simulink model "example_rotor_loop"  (R2016a)
settings: Solver=VariableStepAuto  StartTime=0.0  StopTime=20  RelTol=1e-3
libraries: simulink x2
settings Model: Creator=mgreiff  LastModifiedBy=mgreiff

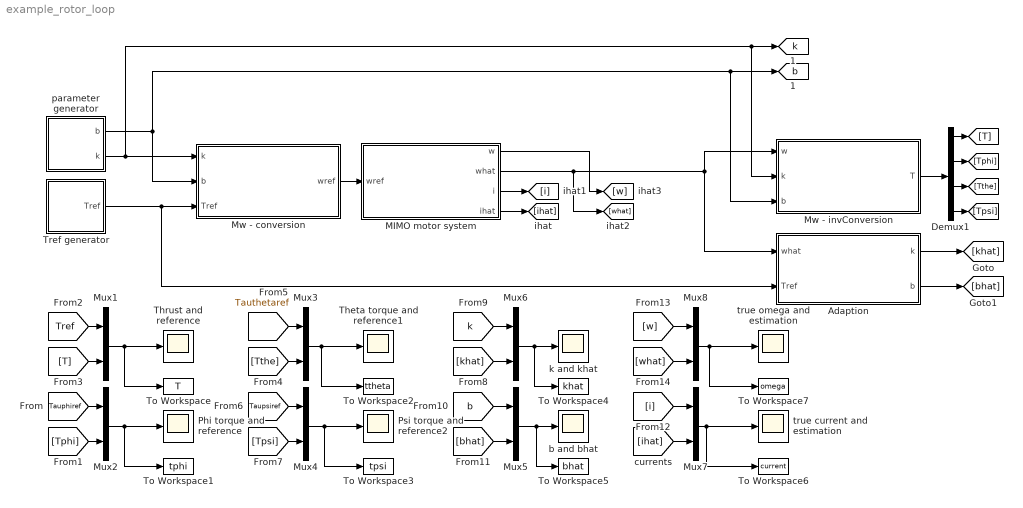
== system example_rotor_loop ==
  Adaption : Subsystem
  Demux1 : Demux
  MIMO motor system : Subsystem
  Mux{1..8} (8 alike) : Mux  Inputs=2
  Mw - conversion : Subsystem
  Mw - invConversion : Subsystem
  Phi torque and reference : Scope
  Psi torque and reference2 : Scope
  Theta torque and reference1 : Scope
  Thrust and reference : Scope
  To Workspace : ToWorkspace  VariableName=T  SaveFormat=Timeseries  SampleTime=-1
  To Workspace1 : ToWorkspace  VariableName=tphi  SaveFormat=Timeseries  SampleTime=-1
  To Workspace2 : ToWorkspace  VariableName=ttheta  SaveFormat=Timeseries  SampleTime=-1
  To Workspace3 : ToWorkspace  VariableName=tpsi  SaveFormat=Timeseries  SampleTime=-1
  To Workspace4 : ToWorkspace  VariableName=khat  SaveFormat=Timeseries  SampleTime=-1
  To Workspace5 : ToWorkspace  VariableName=bhat  SaveFormat=Timeseries  SampleTime=-1
  To Workspace6 : ToWorkspace  VariableName=current  SaveFormat=Timeseries  SampleTime=-1
  To Workspace7 : ToWorkspace  VariableName=omega  SaveFormat=Timeseries  SampleTime=-1
  Tref generator : Subsystem
  b and bhat : Scope
  k and khat : Scope
  parameter generator : Subsystem
  true current and estimation : Scope
  true omega and estimation : Scope
  tag scope: b=global, k=global
  wires:
  MIMO motor system/2(what) -> [what], Adaption/1(what), Mw - invConversion/1(w)
  Mw - conversion/1(wref) -> MIMO motor system/1(wref)
  Tref generator/1(Tref) -> Adaption/2(Tref), Mw - conversion/3(Tref)
  MIMO motor system/3(i) -> [i]
  Mw - invConversion/1(T) -> Demux1/1
  [Tref] -> Mux1/1
  [T] -> Mux1/2
  Mux1/1 -> To Workspace/1, Thrust and reference/1
  Demux1/1 -> [T]
  Demux1/2 -> [Tphi]
  Demux1/3 -> [Tthe]
  Demux1/4 -> [Tpsi]
  [Tauphiref] -> Mux2/1
  [Tphi] -> Mux2/2
  Mux2/1 -> To Workspace1/1, Phi torque and reference/1
  [Tauthetaref] -> Mux3/1
  [Tthe] -> Mux3/2
  Mux3/1 -> To Workspace2/1, Theta torque and reference1/1
  [Taupsiref] -> Mux4/1
  [Tpsi] -> Mux4/2
  Mux4/1 -> Psi torque and reference2/1, To Workspace3/1
  [k] -> Mux6/1
  [khat] -> Mux6/2
  Mux6/1 -> To Workspace4/1, k and khat/1
  [b] -> Mux5/1
  [bhat] -> Mux5/2
  parameter generator/2(k) -> Mw - invConversion/2(k), [k], Mw - conversion/1(k)
  parameter generator/1("b ") -> Mw - conversion/2(b), Mw - invConversion/3(b), [b]
  Adaption/1(k) -> [khat]
  Adaption/2(b) -> [bhat]
  Mux5/1 -> To Workspace5/1, b and bhat/1
  MIMO motor system/4(ihat) -> [ihat]
  [ihat] -> Mux7/2
  [i] -> Mux7/1
  Mux7/1 -> To Workspace6/1, true current and estimation/1
  Mux8/1 -> true omega and estimation/1, To Workspace7/1
  [w] -> Mux8/1
  [what] -> Mux8/2
  MIMO motor system/1(w) -> [w]

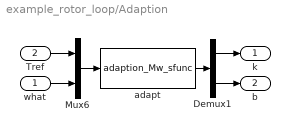
== system example_rotor_loop/Adaption ==
  what : Inport
  Tref : Inport  Port=2
  Demux1 : Demux  Outputs=2
  Mux6 : Mux  Inputs=2
  adapt : S-Function  FunctionName=adaption_Mw_sfunc  SFunctionDeploymentMode=off  EnableBusSupport=off
  k : Outport  PortDimensions=1
  b : Outport  Port=2  PortDimensions=1
  wires:
  Demux1/1 -> k/1
  what/1 -> Mux6/2
  Demux1/2 -> b/1
  Tref/1 -> Mux6/1
  Mux6/1 -> adapt/1
  adapt/1 -> Demux1/1

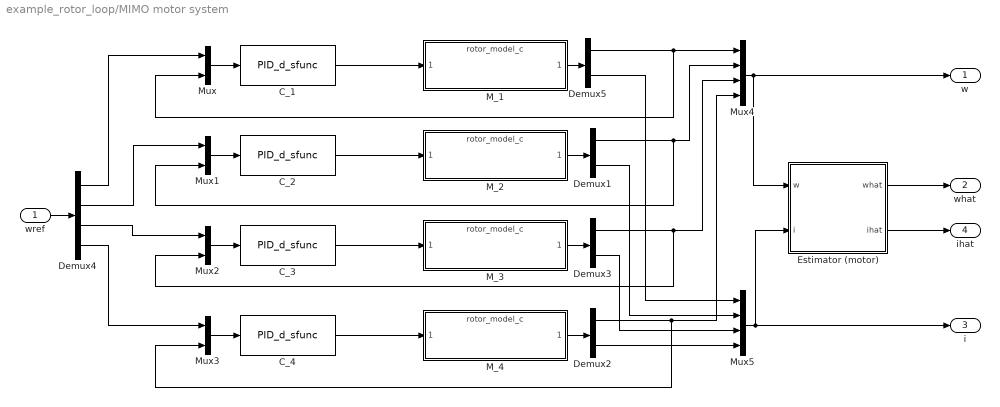
== system example_rotor_loop/MIMO motor system ==
  wref : Inport
  C_{1..4} (4 alike) : S-Function  FunctionName=PID_d_sfunc  Parameters=PIDparam  SFunctionDeploymentMode=off  EnableBusSupport=off
  Demux{1..3,5} (4 alike) : Demux  Outputs=2
  Demux4 : Demux
  Estimator (motor) : Subsystem
  M_{1..4} (4 alike) : ModelReference  ModelNameDialog=rotor_model_c.slx  SimulationMode=Normal  ModelReferenceVersion=1.28
  Mux{,1..3} (4 alike) : Mux  Inputs=2
  Mux4 : Mux
  Mux5 : Mux
  w : Outport
  what : Outport  Port=2
  i : Outport  Port=3
  ihat : Outport  Port=4
  wires:
  Mux1/1 -> C_2/1
  Mux3/1 -> C_4/1
  Demux1/2 -> Mux5/2
  M_4/1 -> Demux2/1
  Demux4/4 -> Mux3/1
  Mux2/1 -> C_3/1
  C_2/1 -> M_2/1
  Demux4/3 -> Mux2/1
  Demux3/1 -> Mux2/2, Mux4/3
  M_2/1 -> Demux1/1
  Mux/1 -> C_1/1
  C_4/1 -> M_4/1
  C_3/1 -> M_3/1
  Demux4/1 -> Mux/1
  Demux3/2 -> Mux5/3
  M_1/1 -> Demux5/1
  Demux4/2 -> Mux1/1
  Demux5/1 -> Mux/2, Mux4/1
  C_1/1 -> M_1/1
  Demux2/2 -> Mux5/4
  M_3/1 -> Demux3/1
  Demux1/1 -> Mux1/2, Mux4/2
  Demux2/1 -> Mux3/2, Mux4/4
  wref/1 -> Demux4/1
  Mux4/1 -> Estimator (motor)/1(w), w/1
  Mux5/1 -> Estimator (motor)/2(i), i/1
  Estimator (motor)/1(what) -> what/1
  Demux5/2 -> Mux5/1
  Estimator (motor)/2(ihat) -> ihat/1

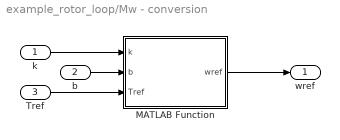
== system example_rotor_loop/Mw - conversion ==
  k : Inport
  b : Inport  Port=2
  Tref : Inport  Port=3
  MATLAB Function : MATLAB Function  TreatAsAtomicUnit=on
  wref : Outport
  wires:
  k/1 -> MATLAB Function/1(k)
  Tref/1 -> MATLAB Function/3(Tref)
  MATLAB Function/1(wref) -> wref/1
  b/1 -> MATLAB Function/2(b)

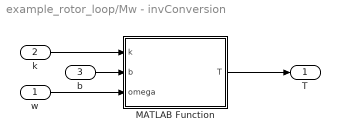
== system example_rotor_loop/Mw - invConversion ==
  w : Inport
  k : Inport  Port=2
  b : Inport  Port=3
  MATLAB Function : MATLAB Function  TreatAsAtomicUnit=on
  T : Outport
  wires:
  k/1 -> MATLAB Function/1(k)
  w/1 -> MATLAB Function/3(omega)
  MATLAB Function/1(T) -> T/1
  b/1 -> MATLAB Function/2(b)

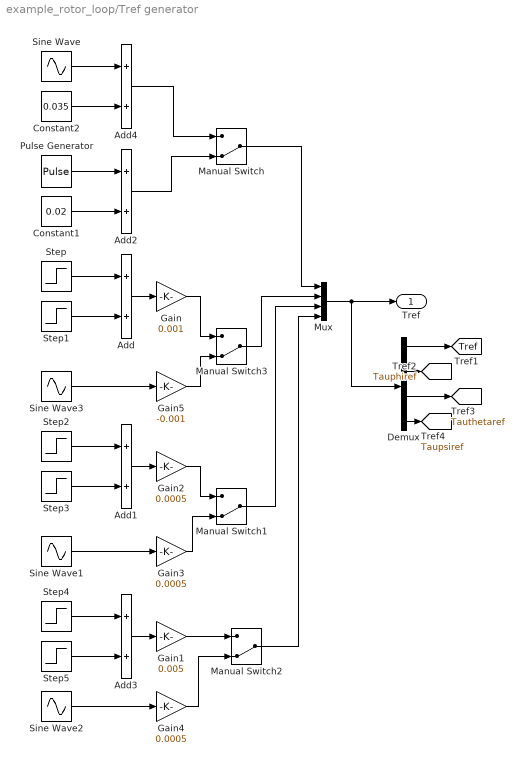
== system example_rotor_loop/Tref generator ==
  Add{,1..4} (5 alike) : Sum
  Constant1 : Constant  Value=0.02
  Constant2 : Constant  Value=0.035
  Demux : Demux
  Gain : Gain  Gain=0.001
  Gain1 : Gain  Gain=0.005
  Gain2 : Gain  Gain=0.0005
  Gain3 : Gain  Gain=0.0005
  Gain4 : Gain  Gain=0.0005
  Gain5 : Gain  Gain=-0.001
  Manual Switch{,1..3} (4 alike) : ManualSwitch  CurrentSetting=0
  Mux : Mux
  Pulse Generator : DiscretePulseGenerator  PulseType=Time based  Amplitude=0.03  Period=4  PulseWidth=50
  Sine Wave : Sin  Amplitude=0.015  SampleTime=0
  Sine Wave1 : Sin  Amplitude=0.5  SampleTime=0
  Sine Wave2 : Sin  Amplitude=0.5  Frequency=0.5  SampleTime=0
  Sine Wave3 : Sin  Amplitude=0.5  Frequency=2  SampleTime=0
  Step : Step  After=-1  SampleTime=0
  Step1 : Step  Time=2  SampleTime=0
  Step2 : Step  Time=4  SampleTime=0
  Step3 : Step  Time=8  After=-1  SampleTime=0
  Step4 : Step  Time=10  SampleTime=0
  Step5 : Step  Time=12  After=-1  SampleTime=0
  Tref : Outport
  tag scope: Tauphiref=global, Taupsiref=global, Tauthetaref=global, Tref=global
  wires:
  Mux/1 -> Demux/1, Tref/1
  Add/1 -> Gain/1
  Demux/1 -> [Tref]
  Demux/2 -> [Tauphiref]
  Demux/3 -> [Tauthetaref]
  Demux/4 -> [Taupsiref]
  Step1/1 -> Add/2
  Step/1 -> Add/1
  Add1/1 -> Gain2/1
  Step3/1 -> Add1/2
  Step2/1 -> Add1/1
  Pulse Generator/1 -> Add2/1
  Constant1/1 -> Add2/2
  Add3/1 -> Gain1/1
  Step5/1 -> Add3/2
  Step4/1 -> Add3/1
  Sine Wave/1 -> Add4/1
  Constant2/1 -> Add4/2
  Add2/1 -> Manual Switch/2
  Add4/1 -> Manual Switch/1
  Manual Switch/1 -> Mux/1
  Sine Wave1/1 -> Gain3/1
  Gain2/1 -> Manual Switch1/1
  Gain3/1 -> Manual Switch1/2
  Manual Switch1/1 -> Mux/3
  Gain1/1 -> Manual Switch2/1
  Sine Wave2/1 -> Gain4/1
  Manual Switch2/1 -> Mux/4
  Gain4/1 -> Manual Switch2/2
  Gain/1 -> Manual Switch3/1
  Gain5/1 -> Manual Switch3/2
  Manual Switch3/1 -> Mux/2
  Sine Wave3/1 -> Gain5/1

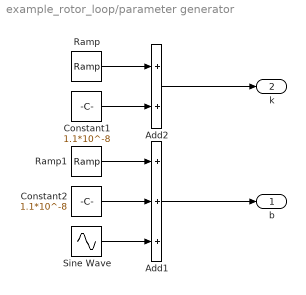
== system example_rotor_loop/parameter generator ==
  Add1 : Sum  Inputs=+++
  Add2 : Sum
  Constant1 : Constant  Value=1.1*10^-8
  Constant2 : Constant  Value=1.1*10^-8
  Ramp : simulink/Sources/Ramp  slope=-10^-10  start=0  X0=0
  Ramp1 : simulink/Sources/Ramp  slope=-10^-10/2  start=0  X0=0
  Sine Wave : Sin  Amplitude=10^-10/2  SampleTime=0
  "b " : Outport  PortDimensions=1
  k : Outport  Port=2  PortDimensions=1
  wires:
  Constant1/1 -> Add2/2
  Ramp/1 -> Add2/1
  Constant2/1 -> Add1/2
  Ramp1/1 -> Add1/1
  Sine Wave/1 -> Add1/3
  Add1/1 -> "b "/1
  Add2/1 -> k/1

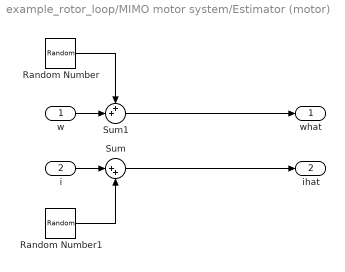
== system example_rotor_loop/MIMO motor system/Estimator (motor) ==
  w : Inport
  i : Inport  Port=2
  Random Number : RandomNumber  Mean=[0,0,0,0]  Variance=20
  Random Number1 : RandomNumber  Mean=[0,0,0,0]  Variance=0.00001
  Sum : Sum  Inputs=|++
  Sum1 : Sum  Inputs=++|
  what : Outport
  ihat : Outport  Port=2
  wires:
  i/1 -> Sum/1
  Sum/1 -> ihat/1
  w/1 -> Sum1/2
  Sum1/1 -> what/1
  Random Number/1 -> Sum1/1
  Random Number1/1 -> Sum/2

== matlab function example_rotor_loop/Mw - invConversion/MATLAB Function ==
  data: k input; b input; T output; omega input
function T = fcn(k, b, omega)
%#codegen
l = 0.1;
omegasq = omega.^2;
Mw = [k   , k   , k  , k  ;
      0   , -k*l, 0  , k*l;
      -k*l, 0   , k*l, 0  ;
      b  , -b   , b , -b  ];
T = Mw*omegasq;

== matlab function example_rotor_loop/Mw - conversion/MATLAB Function ==
  data: k input; b input; wref output; Tref input
function wref = fcn(k, b, Tref)
%#codegen
l = 0.1;
Mw = [1/(4*k), 0         , -1/(2*l*k), 1/(4*b) ;
      1/(4*k), -1/(2*l*k), 0         , -1/(4*b);
      1/(4*k), 0         , 1/(2*l*k) , 1/(4*b) ;
      1/(4*k), 1/(2*l*k) , 0         , -1/(4*b)];
omegasq = Mw * Tref;
wref = sqrt(abs(omegasq));
